simulink subsystem "TRANSFORMATIONS"  (R2025b)
settings: Solver=VariableStepAuto  StartTime=0.0  StopTime=10.0  RelTol=1e-3
model mask{omgCelBod=0}
  mask prompts: omgCelBod "Celestial body angular velocity"
undefined symbols (not defined in the file): simData
libraries: matrix_library x1, simulink_extras x1
settings Model: Creator=antoniohernandez-rodiciomateos  LastModifiedBy=antoniohernandez-rodiciomateos

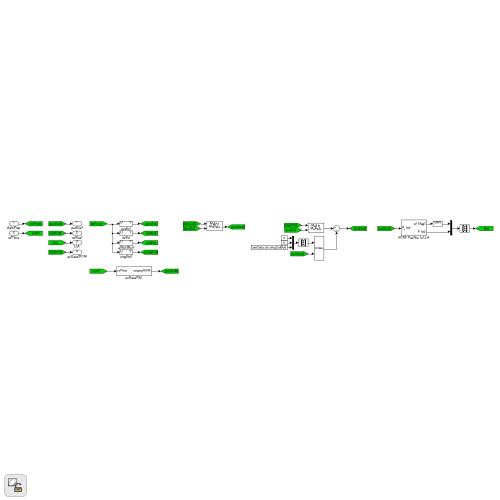
[thumbnail: Simulink's stored preview of the top-level diagram]
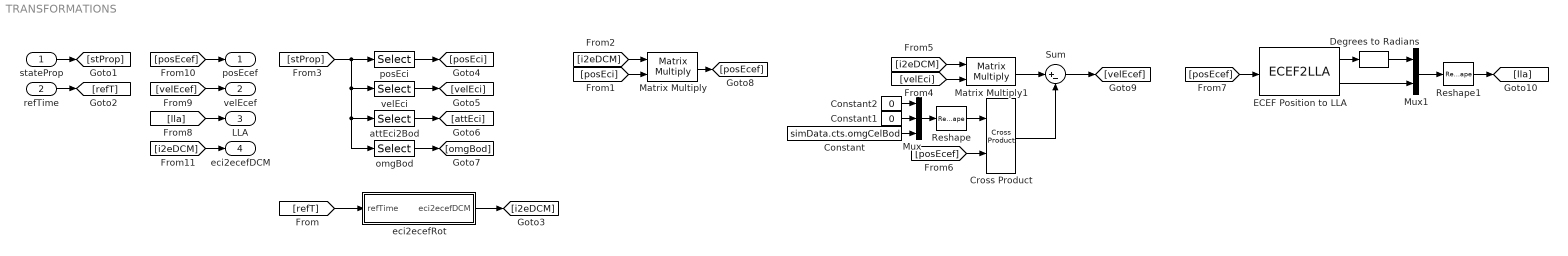
== system TRANSFORMATIONS ==
  stateProp : Inport  PortDimensions=[13 1]
  refTime : Inport  Port=2
  Constant : Constant  Value=simData.cts.omgCelBod
  Constant1 : Constant  Value=0
  Constant2 : Constant  Value=0
  Cross Product : matrix_library/Cross Product
  Degrees to Radians : simulink_extras/Transformations/Degrees to Radians
  ECEF Position to LLA : ECEF2LLA
  Matrix Multiply : Product  Multiplication=Matrix(*)
  Matrix Multiply1 : Product  Multiplication=Matrix(*)
  Mux : Mux  Inputs=3
  Mux1 : Mux  Inputs=2
  Reshape : Reshape  OutputDimensionality=Column vector (2-D)
  Reshape1 : Reshape  OutputDimensionality=Column vector (2-D)
  Sum : Sum  Inputs=|+-
  attEci2Bod : Selector  InputPortWidth=13  IndexOptions=Index vector (dialog)  Indices=[7:10]  OutputSizes=1
  eci2ecefRot : Subsystem
  omgBod : Selector  InputPortWidth=13  IndexOptions=Index vector (dialog)  Indices=[4:6]  OutputSizes=1
  posEci : Selector  InputPortWidth=13  IndexOptions=Index vector (dialog)  Indices=[1:3]  OutputSizes=1
  velEci : Selector  InputPortWidth=13  IndexOptions=Index vector (dialog)  Indices=[4:6]  OutputSizes=1
  posEcef : Outport  PortDimensions=[3 1]
  velEcef : Outport  Port=2
  LLA : Outport  Port=3
  eci2ecefDCM : Outport  Port=4  PortDimensions=[3 3]
  wires:
  stateProp/1 -> [stProp]
  refTime/1 -> [refT]
  [refT] -> eci2ecefRot/1(refTime)
  eci2ecefRot/1(eci2ecefDCM) -> [i2eDCM]
  [stProp] -> omgBod/1, attEci2Bod/1, velEci/1, posEci/1
  posEci/1 -> [posEci]
  velEci/1 -> [velEci]
  attEci2Bod/1 -> [attEci]
  omgBod/1 -> [omgBod]
  [i2eDCM] -> Matrix Multiply/1
  [posEci] -> Matrix Multiply/2
  Matrix Multiply/1 -> [posEcef]
  Constant1/1 -> Mux/2
  Constant2/1 -> Mux/1
  Constant/1 -> Mux/3
  Mux/1 -> Reshape/1
  [velEci] -> Matrix Multiply1/2
  [i2eDCM] -> Matrix Multiply1/1
  Reshape/1 -> Cross Product/1
  [posEcef] -> Cross Product/2
  Matrix Multiply1/1 -> Sum/1
  Cross Product/1 -> Sum/2
  Sum/1 -> [velEcef]
  [posEcef] -> ECEF Position to LLA/1
  [velEcef] -> velEcef/1
  [posEcef] -> posEcef/1
  [lla] -> LLA/1
  [i2eDCM] -> eci2ecefDCM/1
  Degrees to Radians/1 -> Mux1/1
  ECEF Position to LLA/1 -> Degrees to Radians/1
  ECEF Position to LLA/2 -> Mux1/2
  Mux1/1 -> Reshape1/1
  Reshape1/1 -> [lla]

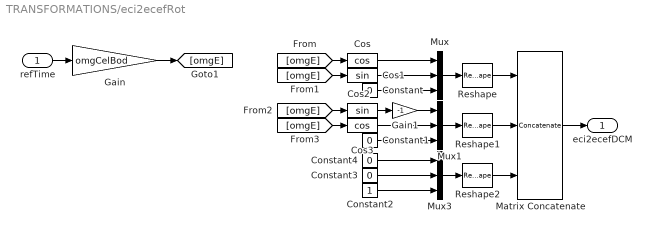
== system TRANSFORMATIONS/eci2ecefRot ==
  refTime : Inport  PortDimensions=[1 1]
  Constant{,1,3..4} (4 alike) : Constant  Value=0
  Constant2 : Constant
  Cos : Trigonometry  Operator=cos
  Cos1 : Trigonometry
  Cos2 : Trigonometry
  Cos3 : Trigonometry  Operator=cos
  Gain : Gain  Gain=omgCelBod
  Gain1 : Gain  Gain=-1
  Matrix Concatenate : Concatenate  NumInputs=3  Mode=Multidimensional array
  Mux : Mux  Inputs=3
  Mux1 : Mux  Inputs=3
  Mux3 : Mux  Inputs=3
  Reshape : Reshape  OutputDimensionality=Row vector (2-D)
  Reshape1 : Reshape  OutputDimensionality=Row vector (2-D)
  Reshape2 : Reshape  OutputDimensionality=Row vector (2-D)
  eci2ecefDCM : Outport  PortDimensions=[3 3]
  wires:
  Reshape/1 -> Matrix Concatenate/1
  Cos/1 -> Mux/1
  Constant/1 -> Mux/3
  Cos1/1 -> Mux/2
  Mux/1 -> Reshape/1
  refTime/1 -> Gain/1
  Gain/1 -> [omgE]
  [omgE] -> Cos/1
  [omgE] -> Cos1/1
  Mux1/1 -> Reshape1/1
  Cos3/1 -> Mux1/2
  [omgE] -> Cos3/1
  Constant1/1 -> Mux1/3
  [omgE] -> Cos2/1
  Cos2/1 -> Gain1/1
  Gain1/1 -> Mux1/1
  Constant4/1 -> Mux3/1
  Mux3/1 -> Reshape2/1
  Constant2/1 -> Mux3/3
  Constant3/1 -> Mux3/2
  Reshape1/1 -> Matrix Concatenate/2
  Reshape2/1 -> Matrix Concatenate/3
  Matrix Concatenate/1 -> eci2ecefDCM/1
